simulink model "ModeloPlantaBuenazoCompatible"  (R2016a)
settings: Solver=ode45  StartTime=0.0  StopTime=188  MaxStep=0.01  RelTol=1e-3
libraries: simulink x1
settings Model: Creator=i95sa  LastModifiedBy=i95sa
settings DataIOCC: SaveFormat=StructureWithTime
settings DebuggingCC: FcnCallInpInsideContextMsg=EnableAllAsWarning
settings HardwareCC: ProdWordSize=32  ProdHWDeviceType=Specified
settings ConfigComp: CovSFcnEnable=off

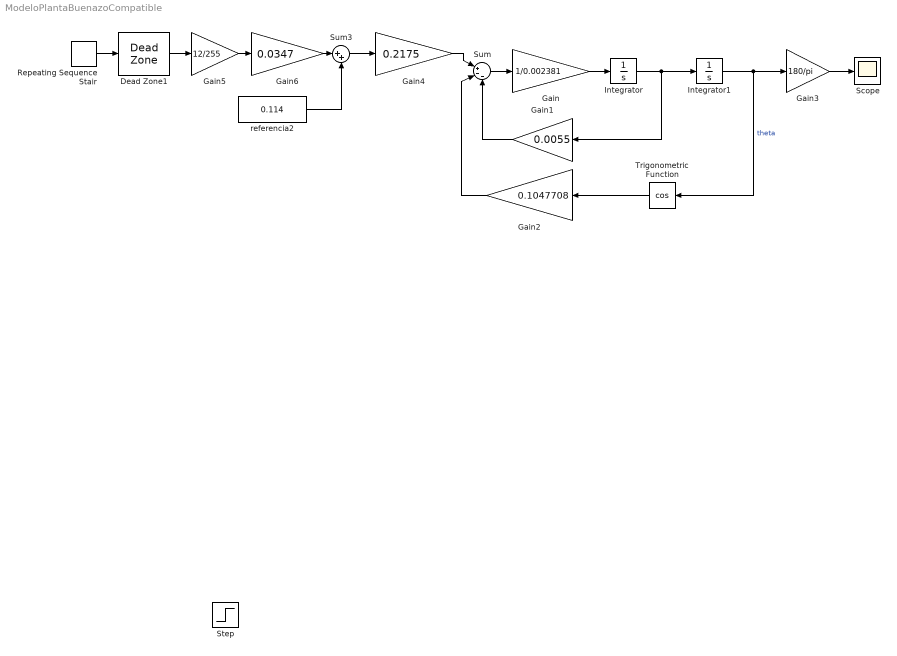
== system ModeloPlantaBuenazoCompatible ==
  Dead Zone1 : DeadZone  LowerValue=0  UpperValue=0  SaturateOnIntegerOverflow=on
  Gain : Gain  Gain=1/0.002381
  Gain1 : Gain  Gain=0.0055
  Gain2 : Gain  Gain=0.1047708
  Gain3 : Gain  Gain=180/pi
  Gain4 : Gain  Gain=0.2175
  Gain5 : Gain  Gain=12/255
  Gain6 : Gain  Gain=0.0347
  Integrator : Integrator
  Integrator1 : Integrator  InitialCondition=-0.65
  Repeating Sequence Stair : simulink/Sources/Repeating Sequence Stair  OutValues=[175 180 185 190 195 200 205 210 215 220 225 230].'  tsamp=17  OutMin=[]  OutMax=[]  OutDataTypeStr=double  OutputDataTypeScalingMode=double  OutDataType=fixdt(0,8)  ConRadixGroup=Best Precision: Vector-wise  OutScaling=2^-12
  Scope : Scope
  Step : Step  Time=0  After=175  SampleTime=0
  Sum : Sum  Inputs=|+--
  Sum3 : Sum  Inputs=|++
  Trigonometric Function : Trigonometry  Operator=cos
  referencia2 : Constant  Value=0.114
  wires:
  Sum/1 -> Gain/1
  Gain/1 -> Integrator/1
  Integrator/1 -> Integrator1/1, Gain1/1
  Trigonometric Function/1 -> Gain2/1
  Gain1/1 -> Sum/3
  Integrator1/1 -> Gain3/1, Trigonometric Function/1  "theta"
  Gain2/1 -> Sum/2
  Gain4/1 -> Sum/1
  referencia2/1 -> Sum3/2
  Sum3/1 -> Gain4/1
  Gain5/1 -> Gain6/1
  Gain6/1 -> Sum3/1
  Dead Zone1/1 -> Gain5/1
  Repeating Sequence Stair/1 -> Dead Zone1/1
  Gain3/1 -> Scope/1
